simulink library "servo_valve_driver_HH_FLO"  (R2025b)
settings: Solver=VariableStepAuto  StartTime=0.0  StopTime=10.0  RelTol=1e-3
libraries: simulink x2, hdlsllib x1, arduinolib x1
settings Model: Creator=cmmcguir  LastModifiedBy=cmmcguir

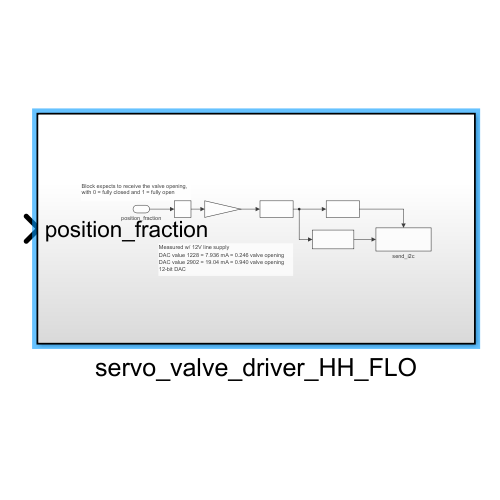
[thumbnail: Simulink's stored preview of the top-level diagram]
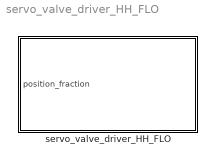
== system servo_valve_driver_HH_FLO ==
  servo_valve_driver_HH_FLO : Subsystem

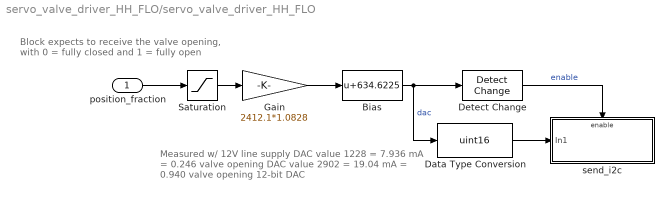
== system servo_valve_driver_HH_FLO/servo_valve_driver_HH_FLO ==
  note: Measured w/ 12V line supply
      | DAC value 1228 = 7.936 mA = 0.246 valve opening
      | DAC value 2902 = 19.04 mA = 0.940 valve opening
      | 12-bit DAC
  note: Block expects to receive the valve opening, with 0 = fully closed and 1 = fully open
  position_fraction : Inport
  Bias : Bias  Bias=634.6225  SaturateOnIntegerOverflow=off
  Data Type Conversion : DataTypeConversion  OutDataTypeStr=uint16  SaturateOnIntegerOverflow=off  RndMeth=Floor
  Detect Change : simulink/Logic and Bit Operations/Detect Change  vinit=0  OutDataTypeStr=boolean
  Gain : Gain  Gain=2412.1*1.0828
  Saturation : Saturate  UpperLimit=1  LowerLimit=0  ZeroCross=off
  send_i2c : Subsystem  TreatAsAtomicUnit=on
  wires:
  position_fraction/1 -> Saturation/1
  Saturation/1 -> Gain/1
  Gain/1 -> Bias/1
  Bias/1 -> Data Type Conversion/1, Detect Change/1  "dac"
  Detect Change/1 -> send_i2c/Enable  "enable"
  Data Type Conversion/1 -> send_i2c/1(In1)

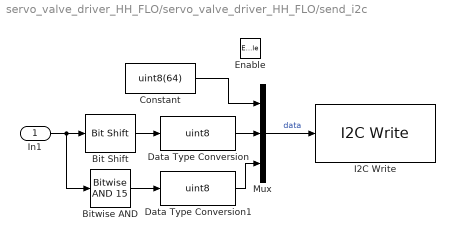
== system servo_valve_driver_HH_FLO/servo_valve_driver_HH_FLO/send_i2c ==
  In1 : Inport
  Enable : EnablePort
  Bit Shift : hdlsllib/Logic and Bit Operations/Bit Shift  mode=Shift Right Logical  N=4
  Bitwise AND : simulink/Logic and Bit Operations/Bitwise Operator  logicop=AND  UseBitMask=on  BitMask=15  BitMaskRealWorld=Stored Integer
      settings: LibrarySourceBlock=|
      | simulink/Quick Insert/Logic and Bit
      | Operations/Bitwise AND
  Constant : Constant  Value=uint8(64)
  Data Type Conversion : DataTypeConversion  OutDataTypeStr=uint8  SaturateOnIntegerOverflow=off  RndMeth=Floor
  Data Type Conversion1 : DataTypeConversion  OutDataTypeStr=uint8  SaturateOnIntegerOverflow=off  RndMeth=Floor
  I2C Write : arduinolib/I2C Write  I2CModule=0  Mode=Master  SlaveAddress=96  SlaveByteOrder=BigEndian  Direction=Transmitter  RegisterAddressMode=off  RegisterAddress=0  SlaveDataType=uint8  DataLength=1  NoAck=off  RepeatedStart=off  OutputStatus=off  blockPlatform=ARDUINO
  Mux : Mux  Inputs=3
  wires:
  Mux/1 -> I2C Write/1  "data"
  Constant/1 -> Mux/1
  Bit Shift/1 -> Data Type Conversion/1
  Data Type Conversion/1 -> Mux/2
  Bitwise AND/1 -> Data Type Conversion1/1
  Data Type Conversion1/1 -> Mux/3
  In1/1 -> Bitwise AND/1, Bit Shift/1
